simulink model "insTestHarness"  (R2024a)
settings: configuration reference "standardSILConfiguraitonParams" (kept outside this file)
settings Model: Creator=aeroth  LastModifiedBy=jerem
settings ConfigSetRef: SourceName=standardSILConfiguraitonParams  SourceLocation=Base Workspace

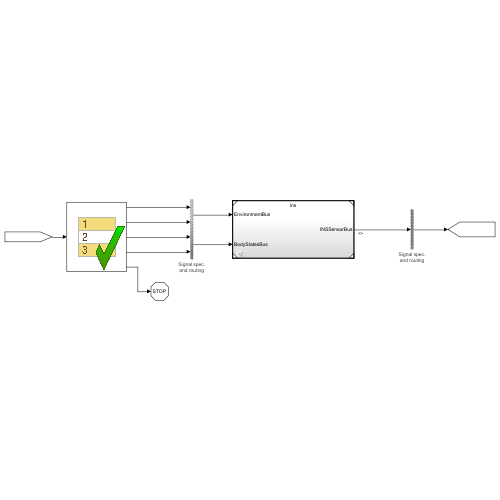
[thumbnail: Simulink's stored preview of the top-level diagram]
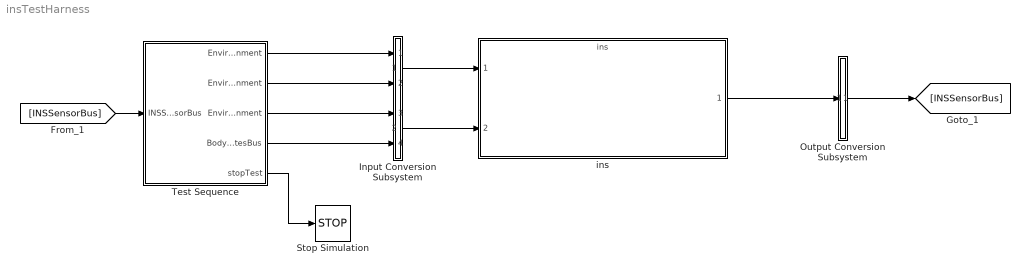
== system insTestHarness ==
  Input Conversion Subsystem : Subsystem  Tag=__SLT_ICS__  Description=|
      | Signal spec.
      | and routing
      settings: AttributesFormatString=%<Description>
  Output Conversion Subsystem : Subsystem  Tag=__SLT_OCS__  Description=|
      | Signal spec.
      | and routing
      mask init:
      | ICDictionary = get_param(bdroot, 'DataDictionary');
      | if isempty(ICDictionary)
      |    ICScope = Simulink.data.BaseWorkspace;
      | else
      |    ICScope = Simulink.data.DataDictionary(ICDictionary);
      | end
      | 
      | IC1 = Simulink.Bus.createMATLABStruct('INSSensorBus', [], [1 1], ICScope);
      settings: AttributesFormatString=%<Description>
  Stop Simulation : Stop
  Test Sequence : Test Sequence  TreatAsAtomicUnit=on
  ins : ModelReference  ModelNameDialog=ins  SimulationMode=Normal  ModelReferenceVersion=1.46
  wires:
  Test Sequence/1(EnvironmentBus_EarthEnvironment) -> Input Conversion Subsystem/1(Inport_1)
  Test Sequence/2(EnvironmentBus_AirEnvironment) -> Input Conversion Subsystem/2(Inport_2)
  Test Sequence/3(EnvironmentBus_TerrainEnvironment) -> Input Conversion Subsystem/3(Inport_3)
  Test Sequence/4(BodyStatesBus) -> Input Conversion Subsystem/4(Inport_4)
  [INSSensorBus] -> Test Sequence/1(INSSensorBus)
  Output Conversion Subsystem/1(Outport_1) -> [INSSensorBus]
  Test Sequence/5(stopTest) -> Stop Simulation/1
  ins/1 -> Output Conversion Subsystem/1(Inport_1)
  Input Conversion Subsystem/1(Outport_1) -> ins/1
  Input Conversion Subsystem/2(Outport_2) -> ins/2

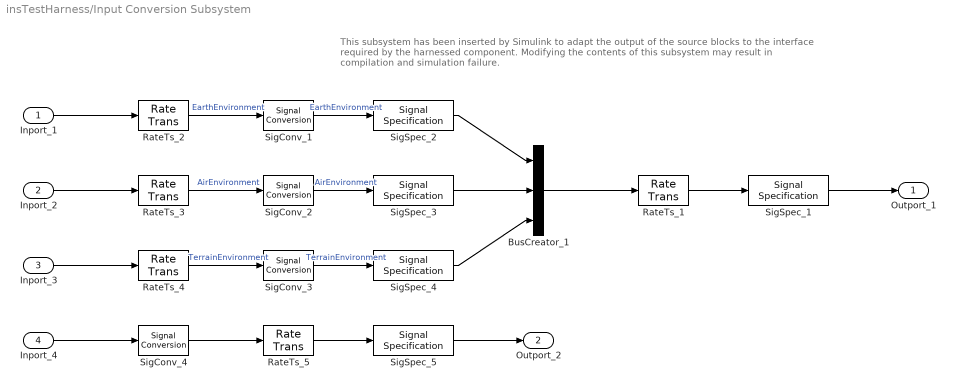
== system insTestHarness/Input Conversion Subsystem ==
  note: This subsystem has been inserted by Simulink to adapt the output of the source blocks to the interface required by the harnessed component.
      |  Modifying the contents of this subsystem may result in compilation and simulation failure.
  Inport_1 : Inport
  Inport_2 : Inport  Port=2
  Inport_3 : Inport  Port=3
  Inport_4 : Inport  Port=4
  BusCreator_1 : BusCreator  Inputs=3  OutDataTypeStr=Bus: EnvironmentBus
  RateTs_{1..5} (5 alike) : RateTransition  OutPortSampleTime=0.004
  SigConv_1 : SignalConversion  ConversionOutput=Nonvirtual bus  OverrideOpt=off
  SigConv_2 : SignalConversion  ConversionOutput=Nonvirtual bus  OverrideOpt=off
  SigConv_3 : SignalConversion  ConversionOutput=Nonvirtual bus  OverrideOpt=off
  SigConv_4 : SignalConversion  ConversionOutput=Virtual bus  OverrideOpt=off
  SigSpec_1 : SignalSpecification  OutDataTypeStr=Bus: EnvironmentBus  SampleTime=0.004
  SigSpec_2 : SignalSpecification  OutDataTypeStr=Bus: EarthEnvironmentBus  Dimensions=[1]  SampleTime=0.004  BusOutputAsStruct=on
  SigSpec_3 : SignalSpecification  OutDataTypeStr=Bus: AirEnvironmentBus  Dimensions=[1]  SampleTime=0.004  BusOutputAsStruct=on
  SigSpec_4 : SignalSpecification  OutDataTypeStr=Bus: TerrainEnvironmentBus  Dimensions=[1]  SampleTime=0.004  BusOutputAsStruct=on
  SigSpec_5 : SignalSpecification  OutDataTypeStr=Bus: BodyStateBus  SampleTime=0.004
  Outport_1 : Outport
  Outport_2 : Outport  Port=2
  wires:
  SigSpec_1/1 -> Outport_1/1
  RateTs_1/1 -> SigSpec_1/1
  BusCreator_1/1 -> RateTs_1/1
  SigSpec_2/1 -> BusCreator_1/1
  SigConv_1/1 -> SigSpec_2/1  "EarthEnvironment"
  RateTs_2/1 -> SigConv_1/1  "EarthEnvironment"
  Inport_1/1 -> RateTs_2/1
  SigSpec_3/1 -> BusCreator_1/2
  SigConv_2/1 -> SigSpec_3/1  "AirEnvironment"
  RateTs_3/1 -> SigConv_2/1  "AirEnvironment"
  Inport_2/1 -> RateTs_3/1
  SigSpec_4/1 -> BusCreator_1/3
  SigConv_3/1 -> SigSpec_4/1  "TerrainEnvironment"
  RateTs_4/1 -> SigConv_3/1  "TerrainEnvironment"
  Inport_3/1 -> RateTs_4/1
  SigSpec_5/1 -> Outport_2/1
  RateTs_5/1 -> SigSpec_5/1
  SigConv_4/1 -> RateTs_5/1
  Inport_4/1 -> SigConv_4/1

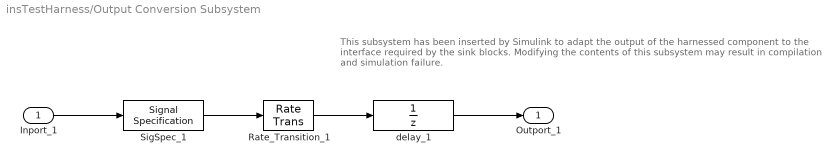
== system insTestHarness/Output Conversion Subsystem ==
  note: This subsystem has been inserted by Simulink to adapt the output of the harnessed component to the interface required by the sink blocks.
      |  Modifying the contents of this subsystem may result in compilation and simulation failure.
  Inport_1 : Inport
  Rate_Transition_1 : RateTransition  OutPortSampleTimeOpt=Inherit
  SigSpec_1 : SignalSpecification  OutDataTypeStr=Bus: INSSensorBus  Dimensions=[1]  SampleTime=0.004
  delay_1 : UnitDelay  InitialCondition=IC1  SampleTime=-1
  Outport_1 : Outport
  wires:
  Inport_1/1 -> SigSpec_1/1
  SigSpec_1/1 -> Rate_Transition_1/1
  Rate_Transition_1/1 -> delay_1/1
  delay_1/1 -> Outport_1/1

== stateflow chart insTestHarness/Test Sequence ==
  state Scenario_1
    state Initialize
      stopTest = false;
      %% Initialize data outputs.
      EnvironmentBus_EarthEnvironment.gravityScalar_mps2 = 9.8;
      %EnvironmentBus_EarthEnvironment.worldMagneticFieldInNED_nT = [40000 0 0]'; %this seems to have no effect
      EnvironmentBus_AirEnvironment.airTemperature_K = 0;
      EnvironmentBus_AirEnvironment.airPressure_Pa = 0;
      EnvironmentBus_AirEnvironment.airDensity_kgpm3 = 0;
      EnvironmentBus_AirEnvironment.windSpeedInNED_mps = zeros(3,1);
      EnvironmentBus_AirEnvironment.speedOfSound_mps = 0;
      EnvironmentBus_TerrainEnvironment.terrainHeightInNED_m = 0;
      BodyStatesBus.aircraftVelInNED_mps = zeros(3,1);
      BodyStatesBus.aircraftPosInNED_m = zeros(3,1);
      BodyStatesBus.aircraftEulerAngles_rad = zeros(3,1);
      BodyStatesBus.aircraftVelInBody_mps = zeros(3,1);
      BodyStatesBus.aircraftAngVelInBody_radps = zeros(3,1);
      BodyStatesBus.aircraftAngAccelInBody_radps2 = zeros(3,1);
      BodyStatesBus.aircraftAccelbe_mps2 = zeros(3,1);
      BodyStatesBus.aircraftAccelInBody_mps2 = zeros(3,1);
      BodyStatesBus.DCM_be = zeros(3,3);
    state checkInsStatic
      verify(isClose(INSSensorBus.GyroSensorBus.x_radps, 0, 'atol', 0.01))
      verify(isClose(INSSensorBus.GyroSensorBus.y_radps, 0, 'atol', 0.01))
      verify(isClose(INSSensorBus.GyroSensorBus.z_radps, 0, 'atol', 0.01))
      %verify(isClose(INSSensorBus.MagSensorBus.x_Gauss, 0)) %TODO something seems off here
      %verify(isClose(INSSensorBus.MagSensorBus.y_Gauss, 0))
      %verify(isClose(INSSensorBus.MagSensorBus.z_Gauss, 0))
      verify(isClose(INSSensorBus.AccelSensorBus.x_mps2, 0, 'atol', 0.01))
      verify(isClose(INSSensorBus.AccelSensorBus.y_mps2, 0, 'atol', 0.01))
      verify(isClose(INSSensorBus.AccelSensorBus.z_mps2, 0, 'atol', 0.01))
    state goInsDynamic
      BodyStatesBus.aircraftVelInNED_mps = zeros(3,1);
      BodyStatesBus.aircraftPosInNED_m = zeros(3,1);
      BodyStatesBus.aircraftEulerAngles_rad = zeros(3,1);
      BodyStatesBus.aircraftVelInBody_mps = zeros(3,1);
      BodyStatesBus.aircraftAngVelInBody_radps = [0.1 0.2 0.3]';
      BodyStatesBus.aircraftAngAccelInBody_radps2 = zeros(3,1);
      BodyStatesBus.aircraftAccelbe_mps2 = [1 2 3]';
      BodyStatesBus.DCM_be = zeros(3,3);
    state checkInsDynamic
      verify(isClose(INSSensorBus.GyroSensorBus.x_radps, 0.1, 'atol', 0.01))
      verify(isClose(INSSensorBus.GyroSensorBus.y_radps, 0.2, 'atol', 0.01))
      verify(isClose(INSSensorBus.GyroSensorBus.z_radps, 0.3, 'atol', 0.01))
      %wtf
      verify(isClose(INSSensorBus.MagSensorBus.x_Gauss, 0, 'atol', 0.01))
      verify(isClose(INSSensorBus.MagSensorBus.y_Gauss, 0, 'atol', 0.01))
      verify(isClose(INSSensorBus.MagSensorBus.z_Gauss, 0, 'atol', 0.01))
      verify(isClose(INSSensorBus.AccelSensorBus.x_mps2, 1, 'atol', 0.01))
      verify(isClose(INSSensorBus.AccelSensorBus.y_mps2, 2, 'atol', 0.01))
      verify(isClose(INSSensorBus.AccelSensorBus.z_mps2, 3, 'atol', 0.01))
    state EndTest
      stopTest = true;
    (default) -> Initialize
    Initialize -> checkInsStatic : [
        | after(5,sec)
        | ]
    checkInsStatic -> goInsDynamic : [
        | true
        | ]
    goInsDynamic -> checkInsDynamic : [
        | after(5,sec)
        | ]
    checkInsDynamic -> EndTest : [
        | true
        | ]
  (default) -> Scenario_1 : {assert(Active_Scenario_Index == 1,'The value of Scenario Parameter ''Active_Scenario_Index'' is not valid. Use the index of the scenario to specify it.')}
  data: INSSensorBus input Bus: INSSensorBus size=[1]; EnvironmentBus_EarthEnvironment output Bus: EarthEnvironmentBus size=[1]; EnvironmentBus_AirEnvironment output Bus: AirEnvironmentBus size=[1]; EnvironmentBus_TerrainEnvironment output Bus: TerrainEnvironmentBus size=[1]; BodyStatesBus output Bus: BodyStateBus size=[1]; Active_Scenario_Index parameter =1; stopTest output
